simulink subsystem "F550_LowFid_Dynamics"  (R2024a)
settings: Solver=VariableStepAuto  StartTime=0.0  StopTime=10.0  RelTol=1e-3
values from neighbouring files (symbols this model uses):
  armLength = 0.275    [F550_data.m]
  dragCoeffMov = 0.01    [F550_data.m]
  g = 9.81    [F550_data.m]
  Mass = 2.06    [F550_data.m]
  motorCr = 1148    [F550_data.m]
  motorRpm0 = [0 0 0 0 0 0]    [F550_data.m]
  motorTm = 0.02    [F550_data.m]
  motorWb = -141.4    [F550_data.m]
  rotorCm = 1.779e-07    [F550_data.m]
  rotorCt = 1.105e-05    [F550_data.m]
  rotorDir = [1 -1 1 -1 -1 1]    [F550_data.m]
  rotorPositions = zeros(3,6)    [F550_data.m]
  rotorThrustMax = 4    [F550_data.m]
  rotorTimeConst = 0.050    (= 0.05)    [F550_data.m]
  rotorTorqueMax = 0.05    [F550_data.m]
  windVel = [0 0 0]'    [F550_data.m]
  x0 = [0 0 0 0 0 0 0 0 0 0 0 0]    [F550_data.m]
undefined symbols (not defined in the file or in its folder): contact, control, ddx, ddy, ddz, dx, dy, dz, earthRadius, p, pitch, q, r, Receive, roll, Send, X, Y, yaw, Z
libraries: aerolibfltsims x3, shared6dof x1, simulink x1, aerolibanimutils x1
settings Model: Creator=CNU_UASG  LastModifiedBy=UASG

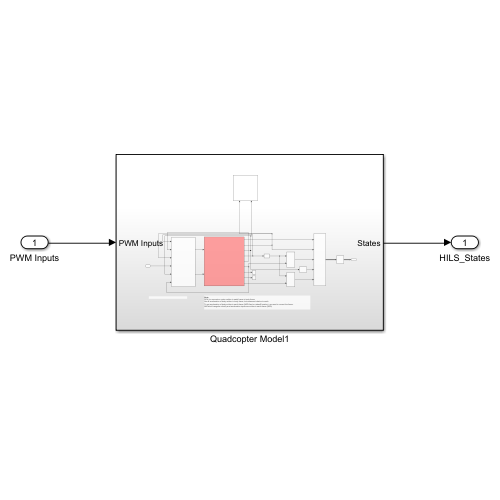
[thumbnail: Simulink's stored preview of the top-level diagram]
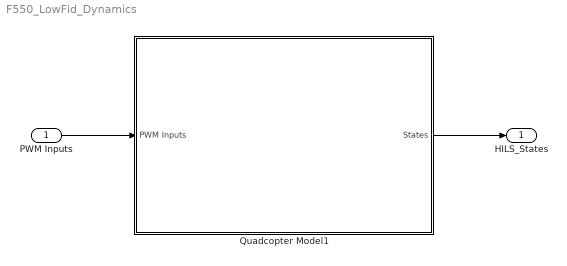
== system F550_LowFid_Dynamics ==
  PWM Inputs : Inport
  Quadcopter Model1 : Subsystem
  HILS_States : Outport
  wires:
  PWM Inputs/1 -> Quadcopter Model1/1(PWM Inputs)
  Quadcopter Model1/1(States) -> HILS_States/1

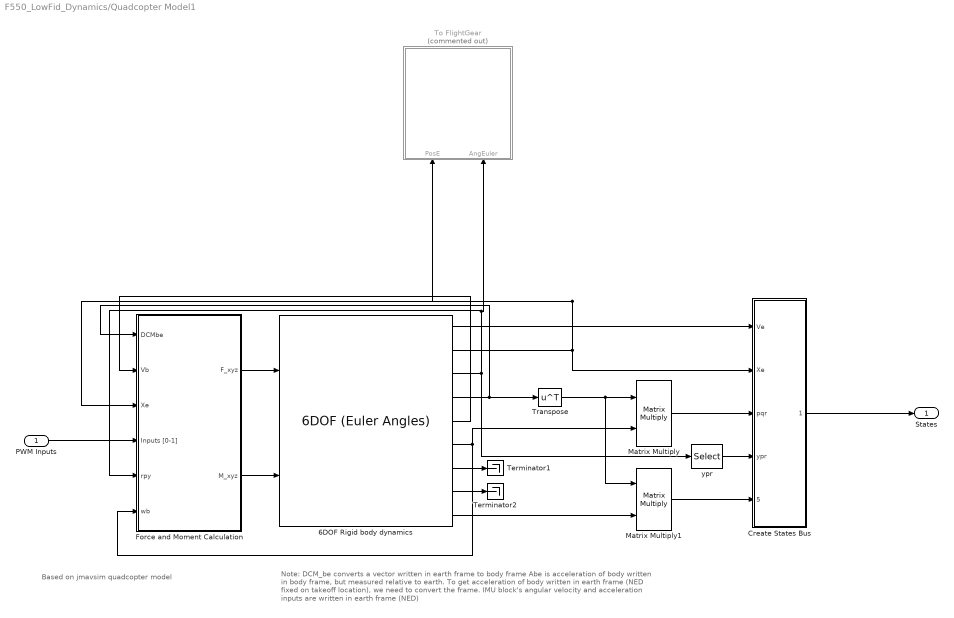
== system F550_LowFid_Dynamics/Quadcopter Model1 ==
  note: Note:
      | DCM_be converts a vector written in earth frame to body frame
      | Abe is acceleration of body written in body frame, but measured relative to earth.
      | To get acceleration of body written in earth frame (NED fixed on takeoff location), we need to convert the frame.
      | IMU block's angular velocity and acceleration inputs are written in earth frame (NED)
  note: Based on jmavsim quadcopter model
  PWM Inputs : Inport
  "6DOF Rigid body dynamics " : shared6dof/6DOF (Euler Angles)  units=Metric (MKS)  mtype=Fixed  rep=Euler Angles  xme_0=x0(10:12)  Vm_0=x0(1:3)  eul_0=x0(7:9)  pm_0=x0(4:6)  mass_0=Mass  mass_e=0.5  mass_f=2.0  inertia=Inertia  inertia_e=eye(3)  inertia_f=2*eye(3)  k_quat=1  vre_flag=on  abi_flag=on  aMode=aMode  xme_statename=''  Vm_statename=''  eul_statename=''  quat_statename=''  pm_statename=''  mass_statename=''
  Create States Bus : Subsystem
  Force and Moment Calculation : Subsystem
  Matrix Multiply : Product  Multiplication=Matrix(*)
  Matrix Multiply1 : Product  Multiplication=Matrix(*)
  Terminator1 : Terminator
  Terminator2 : Terminator
  To FlightGear : Subsystem  Commented=on
      mask Display: image('79904309.png');
  Transpose : Math  Operator=transpose
  ypr : Selector  InputPortWidth=3  IndexOptions=Index vector (dialog)  Indices=[3 2 1]  OutputSizes=1
  States : Outport
  wires:
  PWM Inputs/1 -> Force and Moment Calculation/4(Inputs [0-1])
  Matrix Multiply/1 -> Create States Bus/3(pqr)
  "6DOF Rigid body dynamics "/6 -> Matrix Multiply/2, Force and Moment Calculation/6(wb)
  Force and Moment Calculation/1(F_xyz) -> "6DOF Rigid body dynamics "/1
  "6DOF Rigid body dynamics "/9 -> Matrix Multiply1/2
  Transpose/1 -> Matrix Multiply1/1, Matrix Multiply/1
  "6DOF Rigid body dynamics "/5 -> Force and Moment Calculation/2(Vb)
  ypr/1 -> Create States Bus/4(ypr)
  "6DOF Rigid body dynamics "/2 -> To FlightGear/1(PosE), Force and Moment Calculation/3(Xe), Create States Bus/2(Xe)
  "6DOF Rigid body dynamics "/3 -> To FlightGear/2(AngEuler), Force and Moment Calculation/5(rpy), ypr/1
  Create States Bus/1(States) -> States/1
  "6DOF Rigid body dynamics "/7 -> Terminator1/1
  "6DOF Rigid body dynamics "/1 -> Create States Bus/1(Ve)
  "6DOF Rigid body dynamics "/8 -> Terminator2/1
  Force and Moment Calculation/2(M_xyz) -> "6DOF Rigid body dynamics "/2
  "6DOF Rigid body dynamics "/4 -> Force and Moment Calculation/1(DCMbe), Transpose/1
  Matrix Multiply1/1 -> Create States Bus/5(acc_lnav)

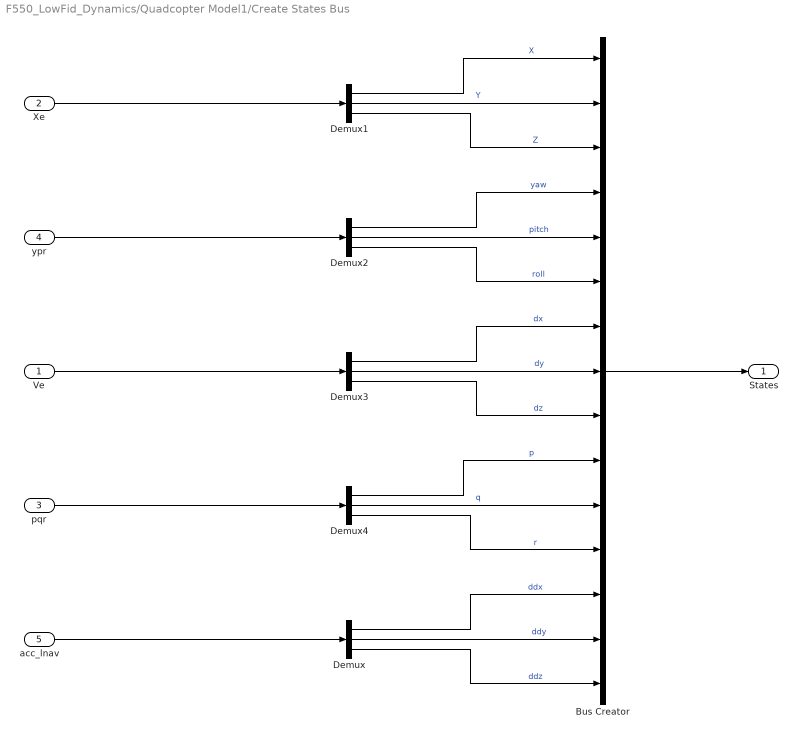
== system F550_LowFid_Dynamics/Quadcopter Model1/Create States Bus ==
  Ve : Inport
  Xe : Inport  Port=2
  pqr : Inport  Port=3
  ypr : Inport  Port=4
  acc_lnav : Inport  Port=5
  Bus Creator : BusCreator  Inputs=X,Y,Z,yaw,pitch,roll,dx,dy,dz,p,q,r,ddx,ddy,ddz
  Demux{,1..4} (5 alike) : Demux  Outputs=3
  States : Outport
  wires:
  Demux1/1 -> Bus Creator/1  "X"
  Demux1/2 -> Bus Creator/2  "Y"
  ypr/1 -> Demux2/1
  Demux2/2 -> Bus Creator/5  "pitch"
  Demux3/2 -> Bus Creator/8  "dy"
  Demux2/3 -> Bus Creator/6  "roll"
  pqr/1 -> Demux4/1
  Ve/1 -> Demux3/1
  Demux2/1 -> Bus Creator/4  "yaw"
  Demux1/3 -> Bus Creator/3  "Z"
  Demux3/1 -> Bus Creator/7  "dx"
  Demux4/2 -> Bus Creator/11  "q"
  Demux3/3 -> Bus Creator/9  "dz"
  Demux4/3 -> Bus Creator/12  "r"
  Demux4/1 -> Bus Creator/10  "p"
  Bus Creator/1 -> States/1
  Xe/1 -> Demux1/1
  acc_lnav/1 -> Demux/1
  Demux/3 -> Bus Creator/15  "ddz"
  Demux/2 -> Bus Creator/14  "ddy"
  Demux/1 -> Bus Creator/13  "ddx"

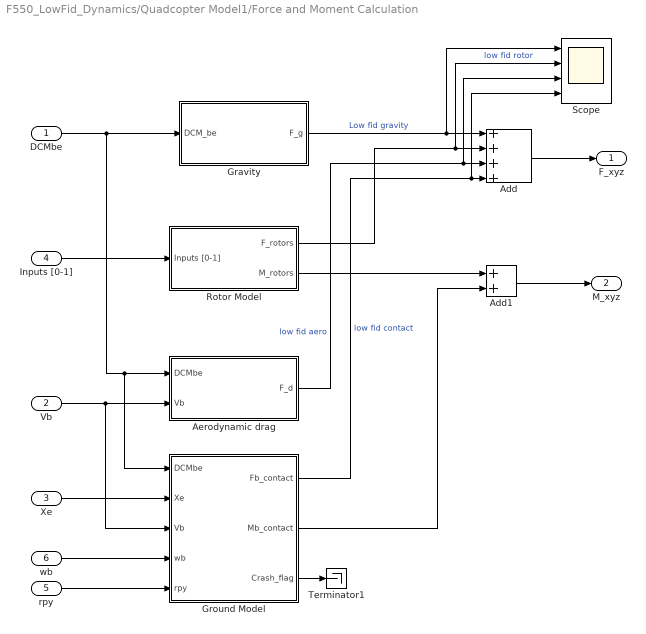
== system F550_LowFid_Dynamics/Quadcopter Model1/Force and Moment Calculation ==
  DCMbe : Inport
  Vb : Inport  Port=2
  Xe : Inport  Port=3
  Inputs [0-1] : Inport  Port=4
  rpy : Inport  Port=5
  wb : Inport  Port=6
  Add : Sum  Inputs=++++
  Add1 : Sum
  Aerodynamic drag : Subsystem
  Gravity : Subsystem
  Ground Model : Subsystem
  Rotor Model : Subsystem
  Scope : Scope  NumInputPorts=4
  Terminator1 : Terminator
  F_xyz : Outport
  M_xyz : Outport  Port=2
  wires:
  Aerodynamic drag/1(F_d) -> Add/3, Scope/3  "low fid aero"
  Inputs [0-1]/1 -> Rotor Model/1(Inputs [0-1])
  DCMbe/1 -> Ground Model/1(DCMbe), Aerodynamic drag/1(DCMbe), Gravity/1(DCM_be)
  Gravity/1(F_g) -> Add/1, Scope/1  "Low fid gravity"
  Add/1 -> F_xyz/1
  Vb/1 -> Ground Model/3(Vb), Aerodynamic drag/2(Vb)
  Rotor Model/1(F_rotors) -> Add/2, Scope/2  "low fid rotor"
  Xe/1 -> Ground Model/2(Xe)
  wb/1 -> Ground Model/4(wb)
  rpy/1 -> Ground Model/5(rpy)
  Rotor Model/2(M_rotors) -> Add1/1
  Ground Model/2(Mb_contact) -> Add1/2
  Add1/1 -> M_xyz/1
  Ground Model/1(Fb_contact) -> Add/4, Scope/4  "low fid contact"
  Ground Model/3(Crash_flag) -> Terminator1/1

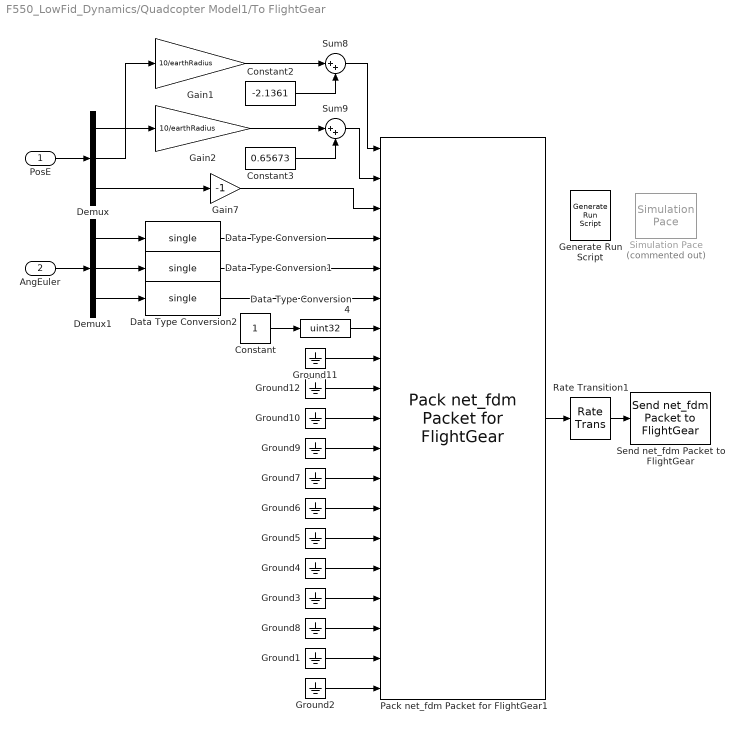
== system F550_LowFid_Dynamics/Quadcopter Model1/To FlightGear ==
  PosE : Inport
  AngEuler : Inport  Port=2
  Constant : Constant
  Constant2 : Constant  Value=-2.1361  VectorParams1D=off
  Constant3 : Constant  Value=0.65673  VectorParams1D=off
  Data Type Conversion : DataTypeConversion  OutDataTypeStr=single  RndMeth=Floor
  Data Type Conversion1 : DataTypeConversion  OutDataTypeStr=single  RndMeth=Floor
  Data Type Conversion2 : DataTypeConversion  OutDataTypeStr=single  RndMeth=Floor
  Data Type Conversion4 : DataTypeConversion  OutDataTypeStr=uint32  SaturateOnIntegerOverflow=off  RndMeth=Floor
  Demux : Demux  Outputs=3
  Demux1 : Demux  Outputs=3
  Gain1 : Gain  Gain=10/earthRadius
  Gain2 : Gain  Gain=10/earthRadius
  Gain7 : Gain  Gain=-1
  Generate Run Script : aerolibfltsims/Generate Run Script  Architecture=Default  dataFlow=Send-Receive  GeometryModelName=Rotor4  AirportId=KSF0  RunwayId=10L  InitialAltitude=0  InitialHeading=0  OffsetDistance=0  OffsetAzimuth=0  InstallScenery=off  DisableShaders=off  OriginAddress=127.0.0.1  DestinationPort=5502  OriginPort=5505  LocalAddress=127.0.0.1  OutputFileName=runfg.bat  FlightGearBaseDirectory=C:\Program Files\FlightGear 2016.1.2
  Ground{1..12} (12 alike) : Ground
  Pack net_fdm Packet for FlightGear1 : aerolibfltsims/Pack net_fdm Packet for FlightGear  FlightGearVersion=v2016.1  ShowPositionAttitudeInputs=on  ShowVelocityAccelerationInputs=off  ShowControlSurfacePositionInputs=off  ShowEngineFuelInputs=on  ShowLandingGearInputs=off  ShowEnvironmentInputs=off  SampleTime=-1  packetVersion=24
  Rate Transition1 : RateTransition
  Send net_fdm Packet to FlightGear : aerolibfltsims/Send net_fdm Packet to FlightGear  DestinationIpAddress=127.0.0.1  DestinationPort=5502  LocalIpPort=-1  varLen=off  SampleTime=0.01
  Simulation Pace : aerolibanimutils/Simulation Pace  Commented=on  SimulationPace=1  SleepMode=MATLAB Thread  OutputPaceError=off  SampleTime=-1
      settings: AttributesFormatString=%<SimulationPace> sec/sec
  Sum8 : Sum  Inputs=|++
  Sum9 : Sum  Inputs=|++
  wires:
  AngEuler/1 -> Demux1/1
  PosE/1 -> Demux/1
  Demux1/1 -> Data Type Conversion/1
  Demux/1 -> Gain2/1
  Constant/1 -> Data Type Conversion4/1
  Demux/3 -> Gain7/1
  Sum9/1 -> Pack net_fdm Packet for FlightGear1/2
  Sum8/1 -> Pack net_fdm Packet for FlightGear1/1
  Data Type Conversion/1 -> Pack net_fdm Packet for FlightGear1/4
  Data Type Conversion1/1 -> Pack net_fdm Packet for FlightGear1/5
  Data Type Conversion2/1 -> Pack net_fdm Packet for FlightGear1/6
  Data Type Conversion4/1 -> Pack net_fdm Packet for FlightGear1/7
  Demux1/2 -> Data Type Conversion1/1
  Pack net_fdm Packet for FlightGear1/1 -> Rate Transition1/1
  Gain2/1 -> Sum9/1
  Gain1/1 -> Sum8/1
  Demux1/3 -> Data Type Conversion2/1
  Demux/2 -> Gain1/1
  Rate Transition1/1 -> Send net_fdm Packet to FlightGear/1
  Constant2/1 -> Sum8/2
  Constant3/1 -> Sum9/2
  Gain7/1 -> Pack net_fdm Packet for FlightGear1/3
  Ground8/1 -> Pack net_fdm Packet for FlightGear1/17
  Ground1/1 -> Pack net_fdm Packet for FlightGear1/18
  Ground2/1 -> Pack net_fdm Packet for FlightGear1/19
  Ground11/1 -> Pack net_fdm Packet for FlightGear1/8
  Ground10/1 -> Pack net_fdm Packet for FlightGear1/10
  Ground9/1 -> Pack net_fdm Packet for FlightGear1/11
  Ground7/1 -> Pack net_fdm Packet for FlightGear1/12
  Ground6/1 -> Pack net_fdm Packet for FlightGear1/13
  Ground5/1 -> Pack net_fdm Packet for FlightGear1/14
  Ground4/1 -> Pack net_fdm Packet for FlightGear1/15
  Ground3/1 -> Pack net_fdm Packet for FlightGear1/16
  Ground12/1 -> Pack net_fdm Packet for FlightGear1/9

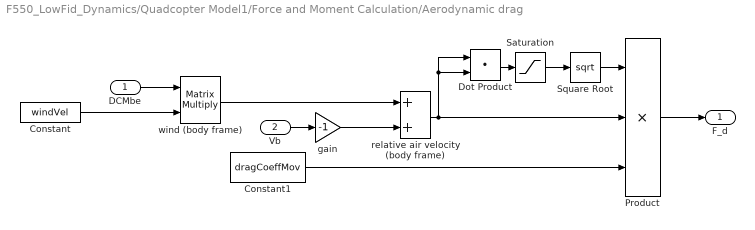
== system F550_LowFid_Dynamics/Quadcopter Model1/Force and Moment Calculation/Aerodynamic drag ==
  DCMbe : Inport
  Vb : Inport  Port=2
  Constant : Constant  Value=windVel
  Constant1 : Constant  Value=dragCoeffMov
  Dot Product : DotProduct  OutDataTypeStr=Inherit: Inherit via internal rule
  Product : Product  Inputs=3
  Saturation : Saturate  UpperLimit=inf  LowerLimit=0.0001
  Square Root : Sqrt
  gain : Gain  Gain=-1
  relative air velocity (body frame) : Sum
  wind (body frame) : Product  Multiplication=Matrix(*)
  F_d : Outport
  wires:
  relative air velocity (body frame)/1 -> Dot Product/2, Dot Product/1, Product/2
  DCMbe/1 -> wind (body frame)/1
  Product/1 -> F_d/1
  Saturation/1 -> Square Root/1
  Vb/1 -> gain/1
  Dot Product/1 -> Saturation/1
  Square Root/1 -> Product/1
  wind (body frame)/1 -> relative air velocity (body frame)/1
  gain/1 -> relative air velocity (body frame)/2
  Constant1/1 -> Product/3
  Constant/1 -> wind (body frame)/2

== system F550_LowFid_Dynamics/Quadcopter Model1/Force and Moment Calculation/Gravity ==
  DCM_be : Inport
  Constant : Constant  Value=[0 0 g]'
  Gain : Gain  Gain=Mass
  Matrix Multiply : Product  Multiplication=Matrix(*)
  F_g : Outport
  wires:
  Matrix Multiply/1 -> Gain/1
  Constant/1 -> Matrix Multiply/2
  DCM_be/1 -> Matrix Multiply/1
  Gain/1 -> F_g/1

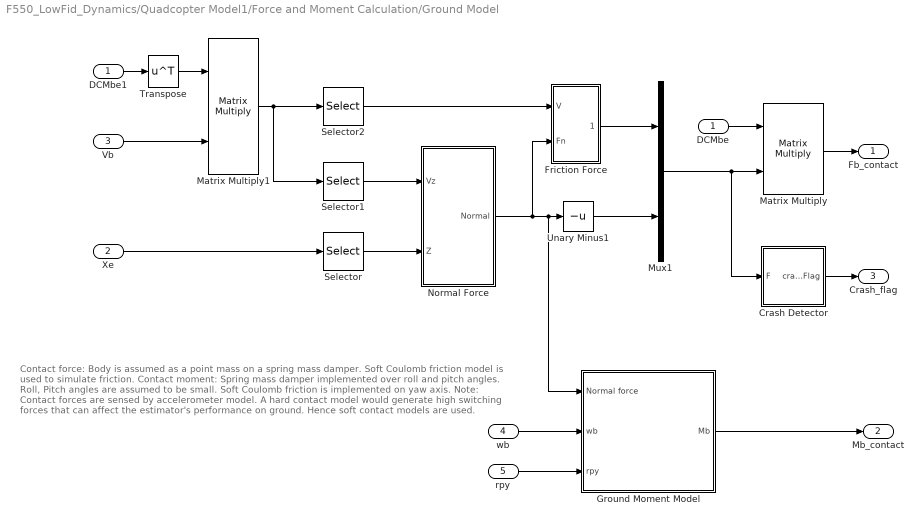
== system F550_LowFid_Dynamics/Quadcopter Model1/Force and Moment Calculation/Ground Model ==
  note: Contact force:
      | Body is assumed as a point mass on a spring mass damper. Soft Coulomb friction model is used to simulate friction.
      |
      | Contact moment:
      | Spring mass damper implemented over roll and pitch angles. Roll, Pitch angles are assumed to be small.
      | Soft Coulomb friction is implemented on yaw axis.
      |
      | Note:
      | Contact forces are sensed by accelerometer model. A hard contact model would generate high switching forces that can affect the estimator's performance on ground. Hence soft contact models are used.
  DCMbe : Inport
  Xe : Inport  Port=2
  Vb : Inport  Port=3
  wb : Inport  Port=4
  rpy : Inport  Port=5
  Crash Detector : Subsystem
  DCMbe1 : InportShadow
  Friction Force : Subsystem
  Ground Moment Model : Subsystem
  Matrix Multiply : Product  Multiplication=Matrix(*)
  Matrix Multiply1 : Product  Multiplication=Matrix(*)
  Mux1 : Mux  Inputs=2
  Normal Force : Subsystem
  Selector : Selector  InputPortWidth=3  IndexOptions=Index vector (dialog)  Indices=[3]  OutputSizes=1
  Selector1 : Selector  InputPortWidth=3  IndexOptions=Index vector (dialog)  Indices=[3]  OutputSizes=1
  Selector2 : Selector  InputPortWidth=3  IndexOptions=Index vector (dialog)  Indices=[1,2]  OutputSizes=1
  Transpose : Math  Operator=transpose
  Unary Minus1 : UnaryMinus
  Fb_contact : Outport
  Mb_contact : Outport  Port=2
  Crash_flag : Outport  Port=3
  wires:
  Crash Detector/1(crashFlag) -> Crash_flag/1
  Xe/1 -> Selector/1
  Selector1/1 -> Normal Force/1(Vz)
  Selector/1 -> Normal Force/2(Z)
  DCMbe/1 -> Matrix Multiply/1
  Matrix Multiply/1 -> Fb_contact/1
  Normal Force/1(Normal) -> Ground Moment Model/1(Normal force), Unary Minus1/1, Friction Force/2(Fn)
  Mux1/1 -> Crash Detector/1(F), Matrix Multiply/2
  Unary Minus1/1 -> Mux1/2
  Selector2/1 -> Friction Force/1(V)
  Friction Force/1(Friction) -> Mux1/1
  DCMbe1/1 -> Transpose/1
  Transpose/1 -> Matrix Multiply1/1
  Vb/1 -> Matrix Multiply1/2
  Matrix Multiply1/1 -> Selector1/1, Selector2/1
  wb/1 -> Ground Moment Model/2(wb)
  rpy/1 -> Ground Moment Model/3(rpy)
  Ground Moment Model/1(Mb) -> Mb_contact/1

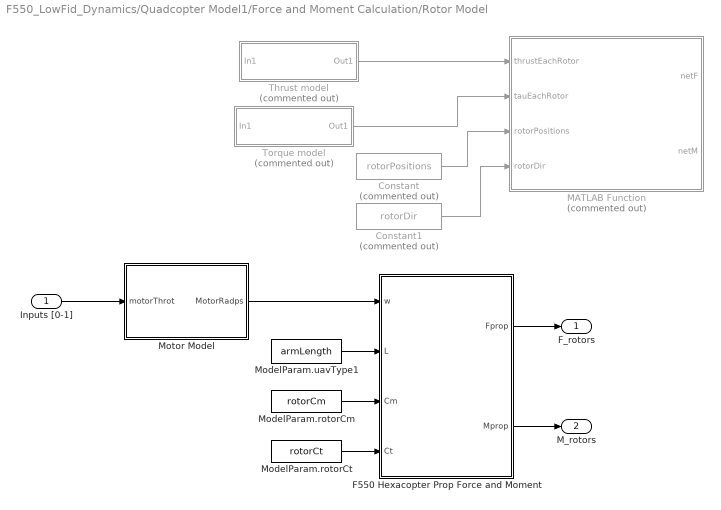
== system F550_LowFid_Dynamics/Quadcopter Model1/Force and Moment Calculation/Rotor Model ==
  Inputs [0-1] : Inport
  Constant : Constant  Commented=on  Value=rotorPositions
  Constant1 : Constant  Commented=on  Value=rotorDir
  F550 Hexacopter Prop Force and Moment : MATLAB Function  TreatAsAtomicUnit=on
  MATLAB Function : MATLAB Function  Commented=on  TreatAsAtomicUnit=on
  ModelParam.rotorCm : Constant  Value=rotorCm
  ModelParam.rotorCt : Constant  Value=rotorCt
  ModelParam.uavType1 : Constant  Value=armLength
  Motor Model : Subsystem
  Thrust model : Subsystem  Commented=on
  Torque model : Subsystem  Commented=on
  F_rotors : Outport
  M_rotors : Outport  Port=2
  wires:
  F550 Hexacopter Prop Force and Moment/2(Mprop) -> M_rotors/1
  F550 Hexacopter Prop Force and Moment/1(Fprop) -> F_rotors/1
  Motor Model/1(MotorRadps) -> F550 Hexacopter Prop Force and Moment/1(w)
  ModelParam.rotorCm/1 -> F550 Hexacopter Prop Force and Moment/3(Cm)
  ModelParam.uavType1/1 -> F550 Hexacopter Prop Force and Moment/2(L)
  ModelParam.rotorCt/1 -> F550 Hexacopter Prop Force and Moment/4(Ct)
  Inputs [0-1]/1 -> Motor Model/1(motorThrot)
  Constant/1 -> MATLAB Function/3(rotorPositions)
  Constant1/1 -> MATLAB Function/4(rotorDir)
  Torque model/1(Out1) -> MATLAB Function/2(tauEachRotor)
  Thrust model/1(Out1) -> MATLAB Function/1(thrustEachRotor)

== system F550_LowFid_Dynamics/Quadcopter Model1/Force and Moment Calculation/Ground Model/Crash Detector ==
  F : Inport
  Compare To Constant : simulink/Logic and Bit Operations/Compare To Constant  relop=>  const=100  OutDataTypeStr=boolean
  Gain : Gain  Gain=1/Mass/g
  norm1 : Subsystem
  crashFlag : Outport
  wires:
  F/1 -> norm1/1(F)
  norm1/1(Out1) -> Gain/1
  Compare To Constant/1 -> crashFlag/1
  Gain/1 -> Compare To Constant/1  "g's"

== system F550_LowFid_Dynamics/Quadcopter Model1/Force and Moment Calculation/Ground Model/Friction Force ==
  V : Inport
  Fn : Inport  Port=2
  Product : Product
  Saturation : Saturate  UpperLimit=contact.translation.maxFriction  LowerLimit=-contact.translation.maxFriction
  Soft Coulomb Friction : Subsystem
  Unary Minus : UnaryMinus
  Friction : Outport
  wires:
  Fn/1 -> Product/2
  Soft Coulomb Friction/1(Out1) -> Product/1
  Product/1 -> Unary Minus/1
  V/1 -> Soft Coulomb Friction/1(In1)
  Unary Minus/1 -> Saturation/1
  Saturation/1 -> Friction/1

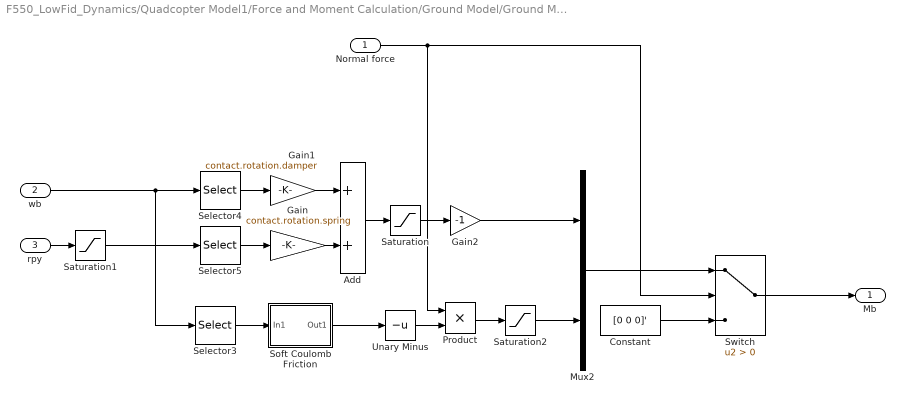
== system F550_LowFid_Dynamics/Quadcopter Model1/Force and Moment Calculation/Ground Model/Ground Moment Model ==
  Normal force : Inport
  wb : Inport  Port=2
  rpy : Inport  Port=3
  Add : Sum
  Constant : Constant  Value=[0 0 0]'
  Gain : Gain  Gain=contact.rotation.spring
  Gain1 : Gain  Gain=contact.rotation.damper
  Gain2 : Gain  Gain=-1
  Mux2 : Mux  Inputs=2
  Product : Product
  Saturation : Saturate  UpperLimit=control.rotation.maxMoment  LowerLimit=-control.rotation.maxMoment
  Saturation1 : Saturate  UpperLimit=20*pi/180  LowerLimit=-20*pi/180
  Saturation2 : Saturate  UpperLimit=control.rotation.maxMoment  LowerLimit=-control.rotation.maxMoment
  Selector3 : Selector  InputPortWidth=3  IndexOptions=Index vector (dialog)  Indices=[3]  OutputSizes=1
  Selector4 : Selector  InputPortWidth=3  IndexOptions=Index vector (dialog)  Indices=[1, 2]  OutputSizes=1
  Selector5 : Selector  InputPortWidth=3  IndexOptions=Index vector (dialog)  Indices=[1, 2]  OutputSizes=1
  Soft Coulomb Friction : Subsystem
  Switch : Switch  Criteria=u2 > Threshold  SaturateOnIntegerOverflow=off  InputSameDT=off
  Unary Minus : UnaryMinus
  Mb : Outport
  wires:
  Gain2/1 -> Mux2/1
  Add/1 -> Saturation/1
  Gain/1 -> Add/2
  Saturation/1 -> Gain2/1
  Selector4/1 -> Gain1/1
  Gain1/1 -> Add/1
  Constant/1 -> Switch/3
  Selector5/1 -> Gain/1
  Switch/1 -> Mb/1
  Mux2/1 -> Switch/1
  Normal force/1 -> Product/1, Switch/2
  rpy/1 -> Saturation1/1
  Saturation1/1 -> Selector5/1
  wb/1 -> Selector4/1, Selector3/1
  Selector3/1 -> Soft Coulomb Friction/1(In1)
  Soft Coulomb Friction/1(Out1) -> Unary Minus/1
  Unary Minus/1 -> Product/2
  Product/1 -> Saturation2/1
  Saturation2/1 -> Mux2/2

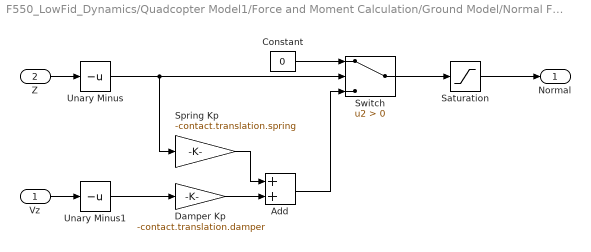
== system F550_LowFid_Dynamics/Quadcopter Model1/Force and Moment Calculation/Ground Model/Normal Force ==
  Vz : Inport
  Z : Inport  Port=2
  Add : Sum
  Constant : Constant  Value=0
  Damper Kp : Gain  Gain=-contact.translation.damper
  Saturation : Saturate  UpperLimit=contact.translation.maxNormal  LowerLimit=0
  Spring Kp : Gain  Gain=-contact.translation.spring
  Switch : Switch  Criteria=u2 > Threshold  SaturateOnIntegerOverflow=off  InputSameDT=off
  Unary Minus : UnaryMinus
  Unary Minus1 : UnaryMinus
  Normal : Outport
  wires:
  Constant/1 -> Switch/1
  Z/1 -> Unary Minus/1
  Switch/1 -> Saturation/1
  Damper Kp/1 -> Add/2
  Add/1 -> Switch/3
  Spring Kp/1 -> Add/1
  Vz/1 -> Unary Minus1/1
  Saturation/1 -> Normal/1
  Unary Minus/1 -> Spring Kp/1, Switch/2
  Unary Minus1/1 -> Damper Kp/1

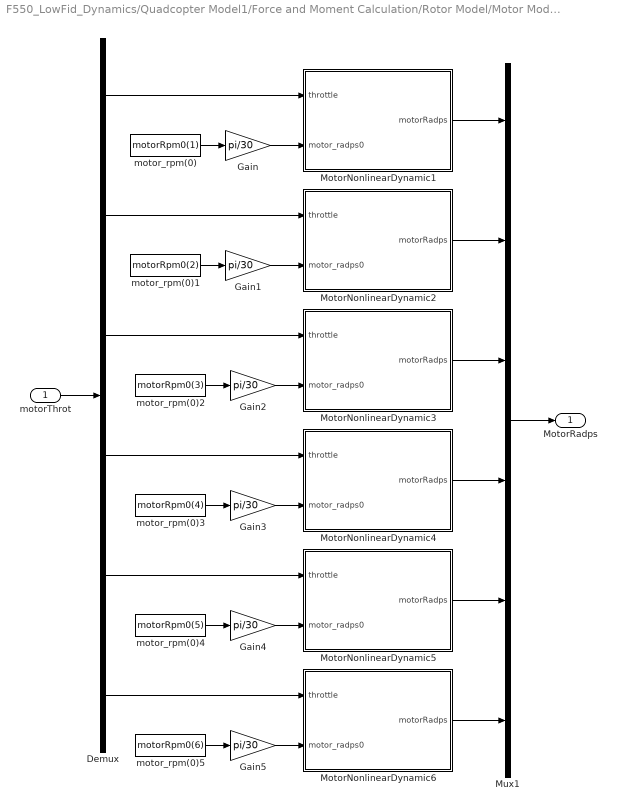
== system F550_LowFid_Dynamics/Quadcopter Model1/Force and Moment Calculation/Rotor Model/Motor Model ==
  motorThrot : Inport
  Demux : Demux  Outputs=6
  Gain{,1..5} (6 alike) : Gain  Gain=pi/30
  MotorNonlinearDynamic1 : Subsystem  TreatAsAtomicUnit=on
  MotorNonlinearDynamic2 : Subsystem  TreatAsAtomicUnit=on
  MotorNonlinearDynamic3 : Subsystem  TreatAsAtomicUnit=on
  MotorNonlinearDynamic4 : Subsystem  TreatAsAtomicUnit=on
  MotorNonlinearDynamic5 : Subsystem  TreatAsAtomicUnit=on
  MotorNonlinearDynamic6 : Subsystem  TreatAsAtomicUnit=on
  Mux1 : Mux  Inputs=6
  motor_rpm(0) : Constant  Value=motorRpm0(1)
  motor_rpm(0)1 : Constant  Value=motorRpm0(2)
  motor_rpm(0)2 : Constant  Value=motorRpm0(3)
  motor_rpm(0)3 : Constant  Value=motorRpm0(4)
  motor_rpm(0)4 : Constant  Value=motorRpm0(5)
  motor_rpm(0)5 : Constant  Value=motorRpm0(6)
  MotorRadps : Outport  VectorParamsAs1DForOutWhenUnconnected=off
  wires:
  motorThrot/1 -> Demux/1
  Demux/4 -> MotorNonlinearDynamic4/1(throttle)
  motor_rpm(0)/1 -> Gain/1
  MotorNonlinearDynamic3/1(motorRadps) -> Mux1/3
  MotorNonlinearDynamic2/1(motorRadps) -> Mux1/2
  Mux1/1 -> MotorRadps/1
  Demux/2 -> MotorNonlinearDynamic2/1(throttle)
  Demux/3 -> MotorNonlinearDynamic3/1(throttle)
  Demux/1 -> MotorNonlinearDynamic1/1(throttle)
  MotorNonlinearDynamic4/1(motorRadps) -> Mux1/4
  MotorNonlinearDynamic1/1(motorRadps) -> Mux1/1
  Gain/1 -> MotorNonlinearDynamic1/2(motor_radps0)
  motor_rpm(0)1/1 -> Gain1/1
  Gain1/1 -> MotorNonlinearDynamic2/2(motor_radps0)
  motor_rpm(0)2/1 -> Gain2/1
  Gain2/1 -> MotorNonlinearDynamic3/2(motor_radps0)
  motor_rpm(0)3/1 -> Gain3/1
  Gain3/1 -> MotorNonlinearDynamic4/2(motor_radps0)
  Gain4/1 -> MotorNonlinearDynamic5/2(motor_radps0)
  motor_rpm(0)4/1 -> Gain4/1
  Demux/5 -> MotorNonlinearDynamic5/1(throttle)
  Gain5/1 -> MotorNonlinearDynamic6/2(motor_radps0)
  motor_rpm(0)5/1 -> Gain5/1
  Demux/6 -> MotorNonlinearDynamic6/1(throttle)
  MotorNonlinearDynamic5/1(motorRadps) -> Mux1/5
  MotorNonlinearDynamic6/1(motorRadps) -> Mux1/6

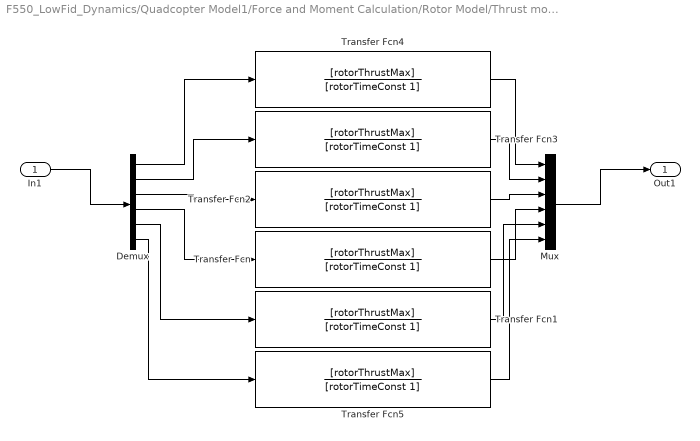
== system F550_LowFid_Dynamics/Quadcopter Model1/Force and Moment Calculation/Rotor Model/Thrust model ==
  In1 : Inport
  Demux : Demux  Outputs=6
  Mux : Mux  Inputs=6
  Transfer Fcn{,1..5} (6 alike) : TransferFcn  Numerator=[rotorThrustMax]  Denominator=[rotorTimeConst 1]
  Out1 : Outport
  wires:
  Transfer Fcn3/1 -> Mux/2
  Demux/1 -> Transfer Fcn4/1
  Transfer Fcn2/1 -> Mux/3
  Demux/3 -> Transfer Fcn2/1
  Mux/1 -> Out1/1
  Transfer Fcn4/1 -> Mux/1
  Demux/4 -> Transfer Fcn/1
  Demux/2 -> Transfer Fcn3/1
  Transfer Fcn/1 -> Mux/4
  In1/1 -> Demux/1
  Demux/5 -> Transfer Fcn1/1
  Demux/6 -> Transfer Fcn5/1
  Transfer Fcn1/1 -> Mux/5
  Transfer Fcn5/1 -> Mux/6

== system F550_LowFid_Dynamics/Quadcopter Model1/Force and Moment Calculation/Rotor Model/Torque model ==
  In1 : Inport
  Demux : Demux  Outputs=6
  Mux : Mux  Inputs=6
  Transfer Fcn{1..6} (6 alike) : TransferFcn  Numerator=[rotorTorqueMax]  Denominator=[rotorTimeConst 1]
  Out1 : Outport
  wires:
  Transfer Fcn4/1 -> Mux/4
  Demux/1 -> Transfer Fcn1/1
  Transfer Fcn3/1 -> Mux/3
  Transfer Fcn2/1 -> Mux/2
  Demux/2 -> Transfer Fcn2/1
  Demux/4 -> Transfer Fcn4/1
  Demux/3 -> Transfer Fcn3/1
  Mux/1 -> Out1/1
  Transfer Fcn1/1 -> Mux/1
  In1/1 -> Demux/1
  Demux/5 -> Transfer Fcn5/1
  Demux/6 -> Transfer Fcn6/1
  Transfer Fcn5/1 -> Mux/5
  Transfer Fcn6/1 -> Mux/6

== system F550_LowFid_Dynamics/Quadcopter Model1/Force and Moment Calculation/Ground Model/Crash Detector/norm1 ==
  F : Inport
  Dot Product : DotProduct  OutDataTypeStr=Inherit: Inherit via internal rule
  Sqrt : Sqrt
  Out1 : Outport
  wires:
  Dot Product/1 -> Sqrt/1
  F/1 -> Dot Product/2, Dot Product/1
  Sqrt/1 -> Out1/1

== system F550_LowFid_Dynamics/Quadcopter Model1/Force and Moment Calculation/Ground Model/Friction Force/Soft Coulomb Friction ==
  note: Pennestrì, E., Rossi, V., Salvini, P. et al. Review and comparison of dry friction force models. Nonlinear Dyn 83, 1785–1801 (2016). https://doi.org/10.1007/s11071-015-2485-3
  In1 : Inport
  Tanh : Trigonometry  Operator=tanh
  friction coefficient : Gain  Gain=contact.translation.friction
  vd : Gain  Gain=1/contact.translation.vd
  Out1 : Outport
  wires:
  In1/1 -> vd/1
  vd/1 -> Tanh/1
  Tanh/1 -> friction coefficient/1
  friction coefficient/1 -> Out1/1

== system F550_LowFid_Dynamics/Quadcopter Model1/Force and Moment Calculation/Ground Model/Ground Moment Model/Soft Coulomb Friction ==
  note: Pennestrì, E., Rossi, V., Salvini, P. et al. Review and comparison of dry friction force models. Nonlinear Dyn 83, 1785–1801 (2016). https://doi.org/10.1007/s11071-015-2485-3
  In1 : Inport
  Tanh : Trigonometry  Operator=tanh
  friction coefficient : Gain  Gain=control.rotation.friction
  vd : Gain  Gain=1/control.rotation.vd
  Out1 : Outport
  wires:
  In1/1 -> vd/1
  vd/1 -> Tanh/1
  Tanh/1 -> friction coefficient/1
  friction coefficient/1 -> Out1/1

== system F550_LowFid_Dynamics/Quadcopter Model1/Force and Moment Calculation/Rotor Model/Motor Model/MotorNonlinearDynamic1 ==
  note: motor throttle 에 따른 motor 회전수 범위는 대략 0~1000 (rad/sec) (=9500rpm)
  throttle : Inport
  motor_radps0 : Inport  Port=2
  Constant : Constant  Value=motorWb
  Gain : Gain  Gain=motorCr
  Motor_Dynamics (1st order) : Subsystem  TreatAsAtomicUnit=on
  Signal_Saturation : Saturate  UpperLimit=0.95  LowerLimit=0
      settings: AttributesFormatString=%<LowerLimit>~%<UpperLimit>
  Sum1 : Sum  Inputs=++|
  motorRadps : Outport  VectorParamsAs1DForOutWhenUnconnected=off
  wires:
  Motor_Dynamics (1st order)/1(motor_radps) -> motorRadps/1
  motor_radps0/1 -> Motor_Dynamics (1st order)/2(motor_radps0)
  Constant/1 -> Sum1/1
  Gain/1 -> Sum1/2
  Signal_Saturation/1 -> Gain/1
  Sum1/1 -> Motor_Dynamics (1st order)/1(motor_radps_cmd)
  throttle/1 -> Signal_Saturation/1

== system F550_LowFid_Dynamics/Quadcopter Model1/Force and Moment Calculation/Rotor Model/Motor Model/MotorNonlinearDynamic2 ==
  note: motor throttle 에 따른 motor 회전수 범위는 대략 0~1000 (rad/sec) (=9500rpm)
  throttle : Inport
  motor_radps0 : Inport  Port=2
  Constant : Constant  Value=motorWb
  Gain : Gain  Gain=motorCr
  Motor_Dynamics (1st order) : Subsystem  TreatAsAtomicUnit=on
  Signal_Saturation : Saturate  UpperLimit=0.95  LowerLimit=0
      settings: AttributesFormatString=%<LowerLimit>~%<UpperLimit>
  Sum1 : Sum  Inputs=++|
  motorRadps : Outport  VectorParamsAs1DForOutWhenUnconnected=off
  wires:
  throttle/1 -> Signal_Saturation/1
  Sum1/1 -> Motor_Dynamics (1st order)/1(motor_radps_cmd)
  Signal_Saturation/1 -> Gain/1
  Gain/1 -> Sum1/2
  Constant/1 -> Sum1/1
  motor_radps0/1 -> Motor_Dynamics (1st order)/2(motor_radps0)
  Motor_Dynamics (1st order)/1(motor_radps) -> motorRadps/1

== system F550_LowFid_Dynamics/Quadcopter Model1/Force and Moment Calculation/Rotor Model/Motor Model/MotorNonlinearDynamic3 ==
  note: motor throttle 에 따른 motor 회전수 범위는 대략 0~1000 (rad/sec) (=9500rpm)
  throttle : Inport
  motor_radps0 : Inport  Port=2
  Constant : Constant  Value=motorWb
  Gain : Gain  Gain=motorCr
  Motor_Dynamics (1st order) : Subsystem  TreatAsAtomicUnit=on
  Signal_Saturation : Saturate  UpperLimit=0.95  LowerLimit=0
      settings: AttributesFormatString=%<LowerLimit>~%<UpperLimit>
  Sum1 : Sum  Inputs=++|
  motorRadps : Outport  VectorParamsAs1DForOutWhenUnconnected=off
  wires:
  Motor_Dynamics (1st order)/1(motor_radps) -> motorRadps/1
  motor_radps0/1 -> Motor_Dynamics (1st order)/2(motor_radps0)
  Constant/1 -> Sum1/1
  Gain/1 -> Sum1/2
  Signal_Saturation/1 -> Gain/1
  Sum1/1 -> Motor_Dynamics (1st order)/1(motor_radps_cmd)
  throttle/1 -> Signal_Saturation/1

== system F550_LowFid_Dynamics/Quadcopter Model1/Force and Moment Calculation/Rotor Model/Motor Model/MotorNonlinearDynamic4 ==
  note: motor throttle 에 따른 motor 회전수 범위는 대략 0~1000 (rad/sec) (=9500rpm)
  throttle : Inport
  motor_radps0 : Inport  Port=2
  Constant : Constant  Value=motorWb
  Gain : Gain  Gain=motorCr
  Motor_Dynamics (1st order) : Subsystem  TreatAsAtomicUnit=on
  Signal_Saturation : Saturate  UpperLimit=0.95  LowerLimit=0
      settings: AttributesFormatString=%<LowerLimit>~%<UpperLimit>
  Sum1 : Sum  Inputs=++|
  motorRadps : Outport  VectorParamsAs1DForOutWhenUnconnected=off
  wires:
  throttle/1 -> Signal_Saturation/1
  Sum1/1 -> Motor_Dynamics (1st order)/1(motor_radps_cmd)
  Signal_Saturation/1 -> Gain/1
  Gain/1 -> Sum1/2
  Constant/1 -> Sum1/1
  motor_radps0/1 -> Motor_Dynamics (1st order)/2(motor_radps0)
  Motor_Dynamics (1st order)/1(motor_radps) -> motorRadps/1

== system F550_LowFid_Dynamics/Quadcopter Model1/Force and Moment Calculation/Rotor Model/Motor Model/MotorNonlinearDynamic5 ==
  note: motor throttle 에 따른 motor 회전수 범위는 대략 0~1000 (rad/sec) (=9500rpm)
  throttle : Inport
  motor_radps0 : Inport  Port=2
  Constant : Constant  Value=motorWb
  Gain : Gain  Gain=motorCr
  Motor_Dynamics (1st order) : Subsystem  TreatAsAtomicUnit=on
  Signal_Saturation : Saturate  UpperLimit=0.95  LowerLimit=0
      settings: AttributesFormatString=%<LowerLimit>~%<UpperLimit>
  Sum1 : Sum  Inputs=++|
  motorRadps : Outport  VectorParamsAs1DForOutWhenUnconnected=off
  wires:
  throttle/1 -> Signal_Saturation/1
  Sum1/1 -> Motor_Dynamics (1st order)/1(motor_radps_cmd)
  Signal_Saturation/1 -> Gain/1
  Gain/1 -> Sum1/2
  Constant/1 -> Sum1/1
  motor_radps0/1 -> Motor_Dynamics (1st order)/2(motor_radps0)
  Motor_Dynamics (1st order)/1(motor_radps) -> motorRadps/1

== system F550_LowFid_Dynamics/Quadcopter Model1/Force and Moment Calculation/Rotor Model/Motor Model/MotorNonlinearDynamic6 ==
  note: motor throttle 에 따른 motor 회전수 범위는 대략 0~1000 (rad/sec) (=9500rpm)
  throttle : Inport
  motor_radps0 : Inport  Port=2
  Constant : Constant  Value=motorWb
  Gain : Gain  Gain=motorCr
  Motor_Dynamics (1st order) : Subsystem  TreatAsAtomicUnit=on
  Signal_Saturation : Saturate  UpperLimit=0.95  LowerLimit=0
      settings: AttributesFormatString=%<LowerLimit>~%<UpperLimit>
  Sum1 : Sum  Inputs=++|
  motorRadps : Outport  VectorParamsAs1DForOutWhenUnconnected=off
  wires:
  throttle/1 -> Signal_Saturation/1
  Sum1/1 -> Motor_Dynamics (1st order)/1(motor_radps_cmd)
  Signal_Saturation/1 -> Gain/1
  Gain/1 -> Sum1/2
  Constant/1 -> Sum1/1
  motor_radps0/1 -> Motor_Dynamics (1st order)/2(motor_radps0)
  Motor_Dynamics (1st order)/1(motor_radps) -> motorRadps/1

== system F550_LowFid_Dynamics/Quadcopter Model1/Force and Moment Calculation/Rotor Model/Motor Model/MotorNonlinearDynamic1/Motor_Dynamics (1st order) ==
  note: radps_dot = (radps_cmd-radps)/Tm
      | or
      | radps/radps_cmd = 1/(Tm*s +1)
  motor_radps_cmd : Inport
  motor_radps0 : Inport  Port=2
  Add : Sum  Inputs=|+-
  Gain : Gain  Gain=1/motorTm
  Integrator : Integrator  InitialConditionSource=external
  motor_radps : Outport  VectorParamsAs1DForOutWhenUnconnected=off
  wires:
  Add/1 -> Gain/1
  motor_radps0/1 -> Integrator/2
  motor_radps_cmd/1 -> Add/1
  Gain/1 -> Integrator/1  "rads_dot"
  Integrator/1 -> Add/2, motor_radps/1  "radps"

== system F550_LowFid_Dynamics/Quadcopter Model1/Force and Moment Calculation/Rotor Model/Motor Model/MotorNonlinearDynamic2/Motor_Dynamics (1st order) ==
  note: radps_dot = (radps_cmd-radps)/Tm
      | or
      | radps/radps_cmd = 1/(Tm*s +1)
  motor_radps_cmd : Inport
  motor_radps0 : Inport  Port=2
  Add : Sum  Inputs=|+-
  Gain : Gain  Gain=1/motorTm
  Integrator : Integrator  InitialConditionSource=external
  motor_radps : Outport  VectorParamsAs1DForOutWhenUnconnected=off
  wires:
  Integrator/1 -> motor_radps/1, Add/2  "radps"
  Gain/1 -> Integrator/1  "rads_dot"
  motor_radps_cmd/1 -> Add/1
  motor_radps0/1 -> Integrator/2
  Add/1 -> Gain/1

== system F550_LowFid_Dynamics/Quadcopter Model1/Force and Moment Calculation/Rotor Model/Motor Model/MotorNonlinearDynamic3/Motor_Dynamics (1st order) ==
  note: radps_dot = (radps_cmd-radps)/Tm
      | or
      | radps/radps_cmd = 1/(Tm*s +1)
  motor_radps_cmd : Inport
  motor_radps0 : Inport  Port=2
  Add : Sum  Inputs=|+-
  Gain : Gain  Gain=1/motorTm
  Integrator : Integrator  InitialConditionSource=external
  motor_radps : Outport  VectorParamsAs1DForOutWhenUnconnected=off
  wires:
  Add/1 -> Gain/1
  motor_radps0/1 -> Integrator/2
  motor_radps_cmd/1 -> Add/1
  Gain/1 -> Integrator/1  "rads_dot"
  Integrator/1 -> Add/2, motor_radps/1  "radps"

== system F550_LowFid_Dynamics/Quadcopter Model1/Force and Moment Calculation/Rotor Model/Motor Model/MotorNonlinearDynamic4/Motor_Dynamics (1st order) ==
  note: radps_dot = (radps_cmd-radps)/Tm
      | or
      | radps/radps_cmd = 1/(Tm*s +1)
  motor_radps_cmd : Inport
  motor_radps0 : Inport  Port=2
  Add : Sum  Inputs=|+-
  Gain : Gain  Gain=1/motorTm
  Integrator : Integrator  InitialConditionSource=external
  motor_radps : Outport  VectorParamsAs1DForOutWhenUnconnected=off
  wires:
  Integrator/1 -> motor_radps/1, Add/2  "radps"
  Gain/1 -> Integrator/1  "rads_dot"
  motor_radps_cmd/1 -> Add/1
  motor_radps0/1 -> Integrator/2
  Add/1 -> Gain/1

== system F550_LowFid_Dynamics/Quadcopter Model1/Force and Moment Calculation/Rotor Model/Motor Model/MotorNonlinearDynamic5/Motor_Dynamics (1st order) ==
  note: radps_dot = (radps_cmd-radps)/Tm
      | or
      | radps/radps_cmd = 1/(Tm*s +1)
  motor_radps_cmd : Inport
  motor_radps0 : Inport  Port=2
  Add : Sum  Inputs=|+-
  Gain : Gain  Gain=1/motorTm
  Integrator : Integrator  InitialConditionSource=external
  motor_radps : Outport  VectorParamsAs1DForOutWhenUnconnected=off
  wires:
  Integrator/1 -> motor_radps/1, Add/2  "radps"
  Gain/1 -> Integrator/1  "rads_dot"
  motor_radps_cmd/1 -> Add/1
  motor_radps0/1 -> Integrator/2
  Add/1 -> Gain/1

== system F550_LowFid_Dynamics/Quadcopter Model1/Force and Moment Calculation/Rotor Model/Motor Model/MotorNonlinearDynamic6/Motor_Dynamics (1st order) ==
  note: radps_dot = (radps_cmd-radps)/Tm
      | or
      | radps/radps_cmd = 1/(Tm*s +1)
  motor_radps_cmd : Inport
  motor_radps0 : Inport  Port=2
  Add : Sum  Inputs=|+-
  Gain : Gain  Gain=1/motorTm
  Integrator : Integrator  InitialConditionSource=external
  motor_radps : Outport  VectorParamsAs1DForOutWhenUnconnected=off
  wires:
  Integrator/1 -> motor_radps/1, Add/2  "radps"
  Gain/1 -> Integrator/1  "rads_dot"
  motor_radps_cmd/1 -> Add/1
  motor_radps0/1 -> Integrator/2
  Add/1 -> Gain/1

== matlab function F550_LowFid_Dynamics/Quadcopter Model1/Force and Moment Calculation/Rotor Model/MATLAB Function ==
  data: thrustEachRotor input; tauEachRotor input; rotorPositions input; netF output; netM output; rotorDir input
function [netF, netM] = getForceMoment(thrustEachRotor, tauEachRotor, rotorPositions, rotorDir)
%#codegen
Fx = 0;
Fy = 0;
Fz = -sum(thrustEachRotor);

netF = [Fx; Fy; Fz];

netM = [0; 0; 0]; %initialize
    for i = 1:6
        rotPos = rotorPositions(:, i);
        Fi = [0, 0, -thrustEachRotor(i)]';
        netM = netM +  cross(rotPos, Fi);%contribution from thrusts of each propeller
        netM(3) = netM(3) - rotorDir(i)*tauEachRotor(i); %contribution from counter torque acting on propeller
    end

end

== matlab function F550_LowFid_Dynamics/Quadcopter Model1/Force and Moment Calculation/Rotor Model/F550 Hexacopter Prop Force and Moment ==
  data: w input; L input; Cm input; Ct input; Fprop output; Mprop output
function [Fprop, Mprop] = fcn(w, L, Cm, Ct)

 % Body Frame : NED Coordinate
 % X-axis : Heading, Y-axis : Right wing, Z-axis : Down

 %  Obtain the force and torque acting on the body. 
 %  The airframe of the hexarotor is as follows: PX4 Hexacopter Configuration
 %     3↓   5↑
 %      \  /
 %   2↑--  -- 1↓
 %      /  \
 %     6↓   4↑
 %  ↑ stands for counterclockwise and ↓stands for clockwise.


 % Input：
 %  w: motor speed，unit：rad/s
 %  L: Arm Length (m) - In case of F550 R = 0.275 m
 %  Cm: torque coefficient
 %  Ct: thrust coefficient
 %  wb: angular velocity in the body coordinate system
 %  Jrp:  moment of inertia of motor rotor + propeller

 % Output:
 %  Fprop: force vector from prop
 %  Mprop: aerodynamic damping moment + gyro moment
        
        % Legacy Code - From F450 Quadcopter 
        %  F_prop = Ct*(w.^2);      % Force from each prop
        %  M_prop = Cm*(w.^2);      % Torque magnitude from each prop
        % 
        %  Fprop = [0; 0; -sum(F_prop)];
        % 
        %  d=sin(pi/4)*R;
        %  Mp= [ d*F_prop'*[-1;  1;  1; -1]
        %        d*F_prop'*[ 1; -1;  1; -1]
        %          M_prop'*[ 1;  1; -1; -1] ];
        % 
        % % gyro moment
        %  M_gyro   = [Jrp*wb(2)*( w(1) + w(2) - w(3) - w(4));  
        %              Jrp*wb(1)*(-w(1) - w(2) + w(3) + w(4));
        %              0];
        % 
        %  Mprop = Mp + M_gyro;
    
    % 로터 회전수에 따른 추력 및 모멘트
    F_prop = Ct * (w.^2);
    M_prop = Cm * (w.^2);
    
    % 프로펠러에 의한 힘 
    Fprop = [0; 0; -sum(F_prop)];
    
    % 로터에 추력/회전에 의해 기체에 작용하는 모멘트
    Mp = [ F_prop'*[-L; L; 0.5*L; -0.5*L; -0.5*L; 0.5*L]
           F_prop'*[0; 0; sqrt(3)/2*L; -sqrt(3)/2*L; sqrt(3)/2*L; -sqrt(3)/2*L]
           M_prop'*[-1; 1; -1; 1; -1; 1;]
         ];
    
    % % 동체 회전에 의해 회전하는 프롭에 작용하는 모멘트
    % M_gyro = [Jrp*wb(2)*( -w(1)+w(2)-w(3)+w(4)-w(5)+w(6) );
    %           -Jrp*wb(1)*( -w(1)+w(2)-w(3)+w(4)-w(5)+w(6));
    %           0;
    %     ];
    
    Mprop = Mp;
end
